simulink subsystem "FrequencyInterpolation"  (R2024a)
settings: Solver=VariableStepAuto  StartTime=0.0  StopTime=10.0  RelTol=1e-3
undefined symbols (not defined in the file or in its folder): osc_sampling_freq, wave_len
settings Model: Creator=dfurodet  LastModifiedBy=david
settings RTWCC: GPUComputeCapability=3.5

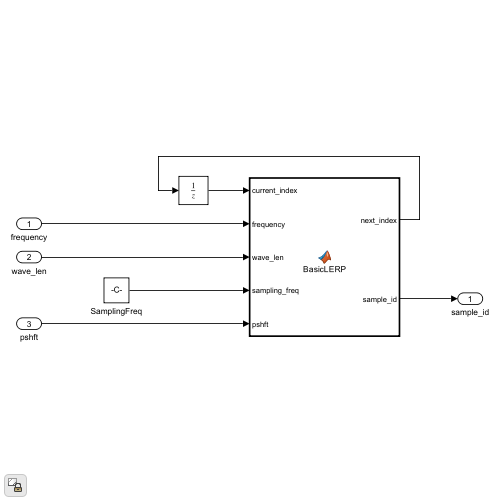
[thumbnail: Simulink's stored preview of the top-level diagram]
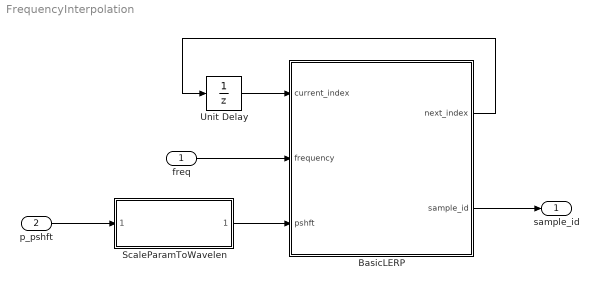
== system FrequencyInterpolation ==
  freq : Inport
  p_pshft : Inport  Port=2
  BasicLERP : MATLAB Function  TreatAsAtomicUnit=on
  ScaleParamToWavelen : Subsystem  ReferencedSubsystem=ScaleParamToWavelen
  Unit Delay : UnitDelay  SampleTime=-1  HasFrameUpgradeWarning=on
  sample_id : Outport  OutDataTypeStr=double
  wires:
  BasicLERP/1(next_index) -> Unit Delay/1
  Unit Delay/1 -> BasicLERP/1(current_index)
  freq/1 -> BasicLERP/2(frequency)
  BasicLERP/2(sample_id) -> sample_id/1
  p_pshft/1 -> ScaleParamToWavelen/1
  ScaleParamToWavelen/1 -> BasicLERP/3(pshft)

== matlab function FrequencyInterpolation/BasicLERP ==
  data: current_index input; next_index output; frequency input; pshft input; sample_id output; osc_sampling_freq parameter; wave_len parameter
function [next_index, sample_id] = BasicLERP(current_index, frequency, pshft, osc_sampling_freq, wave_len)
increment = frequency * wave_len / double(osc_sampling_freq);
next = current_index + increment;
next_index = double(mod(next, wave_len));
sample = current_index + pshft;
sample_id = double(floor(mod(sample, wave_len)));
